simulink model "caishi"  (R2017a)
settings: Solver=FixedStepAuto  StartTime=0.0  StopTime=100  FixedStep=0.001  RelTol=1e-3
values from neighbouring files (symbols this model uses):
  A = [0 1 0 0;0 0 -1 0;0 0 0 1;0 0 22 0]    [keshe6.m]    (also in keshe7.m = [-18/7 9 0;1 -1 1;0 -14.28 0])
  H = [27/7;0;0]    [keshe7.m]
  K = acker(A,B,P)    [keshe6.m]    (also in keshe7.m = inv(Ph)*Vh)
settings Model: Creator=adi  LastModifiedBy=adi

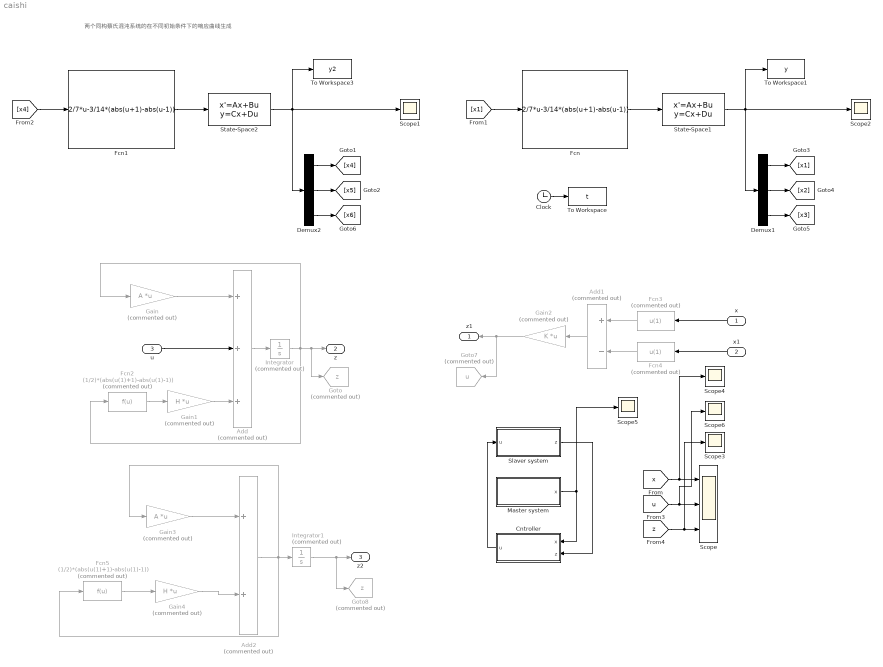
== system caishi ==
  note: 两个同构蔡氏混沌系统的在不同初始条件下的响应曲线生成
  x : Inport
  x1 : Inport  Port=2
  u : Inport  Port=3
  Add : Sum  Commented=on  Inputs=+++
  Add1 : Sum  Commented=on  Inputs=+-
  Add2 : Sum  Commented=on
  Clock : Clock
  Cntroller : Subsystem
  Demux1 : Demux  Outputs=3
  Demux2 : Demux  Outputs=3
  Fcn : Fcn  Expr=2/7*u-3/14*(abs(u+1)-abs(u-1))
  Fcn1 : Fcn  Expr=2/7*u-3/14*(abs(u+1)-abs(u-1))
  Fcn2 : Fcn  Commented=on  Expr=(1/2)*(abs(u(1)+1)-abs(u(1)-1))
  Fcn3 : Fcn  Commented=on  Expr=u(1)
  Fcn4 : Fcn  Commented=on  Expr=u(1)
  Fcn5 : Fcn  Commented=on  Expr=(1/2)*(abs(u(1)+1)-abs(u(1)-1))
  Gain : Gain  Commented=on  Gain=A  Multiplication=Matrix(K*u)
  Gain1 : Gain  Commented=on  Gain=H  Multiplication=Matrix(K*u)
  Gain2 : Gain  Commented=on  Gain=K  Multiplication=Matrix(K*u)
  Gain3 : Gain  Commented=on  Gain=A  Multiplication=Matrix(K*u)
  Gain4 : Gain  Commented=on  Gain=H  Multiplication=Matrix(K*u)
  Goto : Goto  Commented=on  GotoTag=z  TagVisibility=global
  Goto7 : Goto  Commented=on  GotoTag=u  TagVisibility=global
  Goto8 : Goto  Commented=on  GotoTag=z  TagVisibility=global
  Integrator : Integrator  Commented=on  InitialCondition=[0 0 0]
  Integrator1 : Integrator  Commented=on  InitialCondition=[0 0 0]
  Master system : Subsystem
  Scope : Scope  NumInputPorts=3
  Scope{1..6} (6 alike) : Scope
  Slaver system : Subsystem
  State-Space1 : StateSpace  A=[0 9 0;1 -1 1;0 -14.28 0]  B=[-9;0;0]  C=[1 0 0;0 1 0;0 0 1]  D=[0;0;0]  X0=[-0.2;0.3;0.7]
  State-Space2 : StateSpace  A=[0 9 0;1 -1 1;0 -14.28 0]  B=[-9;0;0]  C=[1 0 0;0 1 0;0 0 1]  D=[0;0;0]  X0=[0.2;0.4;0.6]
  To Workspace : ToWorkspace  VariableName=t  SampleTime=-1
  To Workspace1 : ToWorkspace  VariableName=y  SampleTime=-1
  To Workspace3 : ToWorkspace  VariableName=y2  SampleTime=-1
  z1 : Outport
  z : Outport  Port=2
  z2 : Outport  Port=3
  wires:
  Demux1/1 -> [x1]
  [x1] -> Fcn/1
  Clock/1 -> To Workspace/1
  State-Space1/1 -> To Workspace1/1, Scope2/1, Demux1/1
  Demux1/2 -> [x2]
  Demux1/3 -> [x3]
  Fcn/1 -> State-Space1/1
  Demux2/1 -> [x4]
  State-Space2/1 -> To Workspace3/1, Scope1/1, Demux2/1
  Demux2/3 -> [x6]
  [x4] -> Fcn1/1
  Fcn1/1 -> State-Space2/1
  Demux2/2 -> [x5]
  Gain/1 -> Add/1
  u/1 -> Add/2
  Add/1 -> Integrator/1
  Integrator/1 -> Goto/1, z/1, Fcn2/1, Gain/1
  Fcn2/1 -> Gain1/1
  Gain1/1 -> Add/3
  Gain2/1 -> Goto7/1, z1/1
  Add1/1 -> Gain2/1
  Fcn3/1 -> Add1/1
  Fcn4/1 -> Add1/2
  x/1 -> Fcn3/1
  x1/1 -> Fcn4/1
  Fcn5/1 -> Gain4/1
  Integrator1/1 -> Goto8/1, z2/1
  Gain3/1 -> Add2/1
  Gain4/1 -> Add2/2
  Add2/1 -> Fcn5/1, Gain3/1, Integrator1/1
  Cntroller/1(u) -> Slaver system/1(u)
  Slaver system/1(z) -> Cntroller/2(z)
  [z] -> Scope3/1, Scope/3
  [x] -> Scope4/1, Scope/1
  Master system/1(x) -> Scope5/1, Cntroller/1(x)
  [u] -> Scope6/1, Scope/2

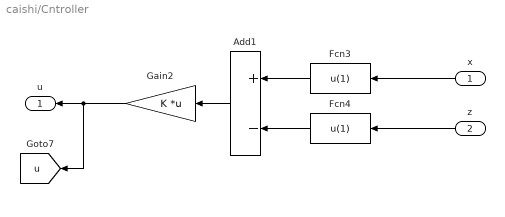
== system caishi/Cntroller ==
  x : Inport
  z : Inport  Port=2
  Add1 : Sum  Inputs=+-
  Fcn3 : Fcn  Expr=u(1)
  Fcn4 : Fcn  Expr=u(1)
  Gain2 : Gain  Gain=K  Multiplication=Matrix(K*u)
  u : Outport
  tag scope: u=global
  wires:
  z/1 -> Fcn4/1
  Fcn3/1 -> Add1/1
  Fcn4/1 -> Add1/2
  Gain2/1 -> [u], u/1
  x/1 -> Fcn3/1
  Add1/1 -> Gain2/1

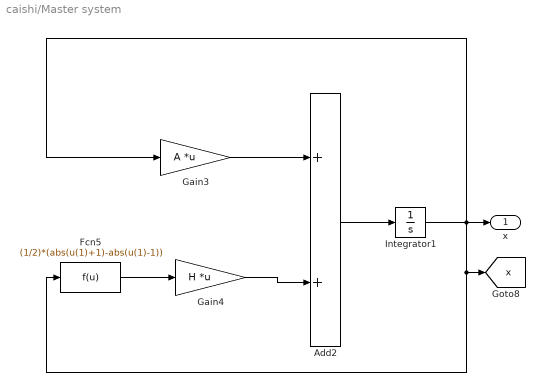
== system caishi/Master system ==
  Add2 : Sum
  Fcn5 : Fcn  Expr=(1/2)*(abs(u(1)+1)-abs(u(1)-1))
  Gain3 : Gain  Gain=A  Multiplication=Matrix(K*u)
  Gain4 : Gain  Gain=H  Multiplication=Matrix(K*u)
  Integrator1 : Integrator  InitialCondition=[0.3 0.3 0.3]
  x : Outport
  tag scope: x=global
  wires:
  Fcn5/1 -> Gain4/1
  Gain4/1 -> Add2/2
  Integrator1/1 -> Fcn5/1, [x], Gain3/1, x/1
  Gain3/1 -> Add2/1
  Add2/1 -> Integrator1/1

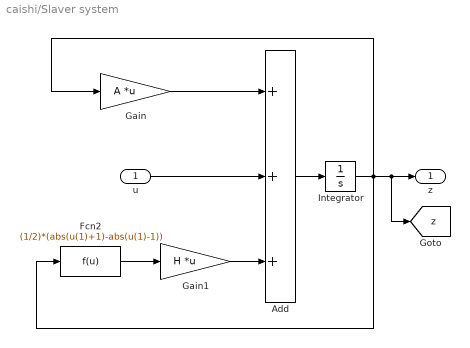
== system caishi/Slaver system ==
  u : Inport
  Add : Sum  Inputs=+++
  Fcn2 : Fcn  Expr=(1/2)*(abs(u(1)+1)-abs(u(1)-1))
  Gain : Gain  Gain=A  Multiplication=Matrix(K*u)
  Gain1 : Gain  Gain=H  Multiplication=Matrix(K*u)
  Integrator : Integrator  InitialCondition=[-0.2 0.3 0.7]
  z : Outport
  tag scope: z=global
  wires:
  Gain1/1 -> Add/3
  Add/1 -> Integrator/1
  Integrator/1 -> [z], z/1, Fcn2/1, Gain/1
  Fcn2/1 -> Gain1/1
  Gain/1 -> Add/1
  u/1 -> Add/2
